simulink model "NAVI_V1_1"  (R2018a)
settings: Solver=VariableStepAuto  StartTime=0.0  StopTime=10.0  FixedStep=sampletime  RelTol=1e-3  EnableMultiTasking=on
PreLoadFcn:
  | NAVI_V1_BusInfo;
libraries: simulink x2
settings Model: Creator=IAEC nishito  LastModifiedBy=nishito
settings DataIOCC: LimitDataPoints=on  SaveFormat=Array  SignalLoggingSaveFormat=ModelDataLogs  SaveOutput=off
settings OptimizationCC: DefaultParameterBehavior=Inlined  ExpressionDepthLimit=2147483647  LifeSpan=inf
settings DebuggingCC: UnderspecifiedInitializationDetection=Classic  MergeDetectMultiDrivingBlocksExec=none  SolverPrmCheckMsg=warning  FcnCallInpInsideContextMsg=warning  StateNameClashWarn=warning  SFUnexpectedBacktrackingDiag=warning  SFNoUnconditionalDefaultTransitionDiag=warning  SFExecutionAtInitializationDiag=none
settings HardwareCC: ProdBitPerPointer=32  ProdBitPerSizeT=32  ProdBitPerPtrDiffT=32  ProdLargestAtomicFloat=None  ProdIntDivRoundTo=Undefined  ProdEndianess=Unspecified  ProdWordSize=32  ProdHWDeviceType=32-bit Generic
settings ModelReferenceCC: UpdateModelReferenceTargets=IfOutOfDate  PropagateSignalLabelsOutOfModel=off
settings CodeAppCC: StateflowObjectComments=on
settings GRTTargetCC: TargetLangStandard=C89/C90 (ANSI)  GeneratePreprocessorConditionals=Disable all  CombineOutputUpdateFcns=off  GRTInterface=on
settings ConfigComp: CovMetricSettings=dw  CovHtmlReporting=on  CovSaveCumulativeToWorkspaceVar=on  CovSaveSingleToWorkspaceVar=on  CovExternalEMLEnable=off  CovSFcnEnable=off

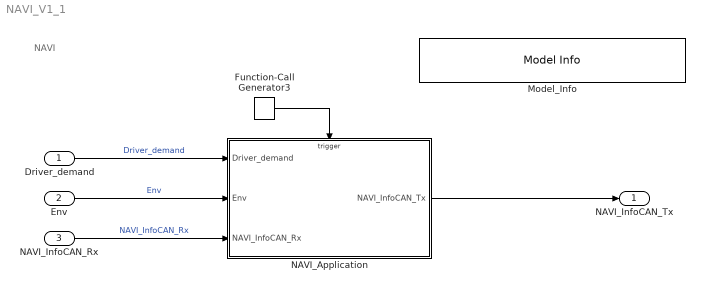
== system NAVI_V1_1 ==
  note: NAVI
  Driver_demand : Inport  OutDataTypeStr=Bus: Driver_demand_Bus
      settings: AttributesFormatString=<%<OutDataTypeStr>>
  Env : Inport  Port=2  OutDataTypeStr=Bus: Environment_Bus
      settings: AttributesFormatString=<%<OutDataTypeStr>>
  NAVI_InfoCAN_Rx : Inport  Port=3  OutDataTypeStr=Bus: NAVI_InfoCAN_Rx_Bus
      settings: AttributesFormatString=<%<OutDataTypeStr>>
  Function-Call Generator3 : simulink/Ports & Subsystems/Function-Call Generator  sample_time=0.1  numberOfIterations=1
      settings: AttributesFormatString=<sample_time=%<sample_time>>
  Model_Info : simulink/Model-Wide Utilities/Model Info  Frame=on  DisplayStringWithTags=|  HorizontalTextAlignment=Left  LeftAlignmentValue=0.02
      | Version  %<ModelVersion>
      | LastModifided by %<LastModifiedBy>  Date %<LastModificationDate>
      | Description  %<Description>
  NAVI_Application : Subsystem
  NAVI_InfoCAN_Tx : Outport  OutDataTypeStr=Bus: NAVI_InfoCAN_Tx_Bus
      settings: AttributesFormatString=<%<OutDataTypeStr>>
  wires:
  NAVI_Application/1(NAVI_InfoCAN_Tx) -> NAVI_InfoCAN_Tx/1
  NAVI_InfoCAN_Rx/1 -> NAVI_Application/3(NAVI_InfoCAN_Rx)  "NAVI_InfoCAN_Rx"
  Driver_demand/1 -> NAVI_Application/1(Driver_demand)  "Driver_demand"
  Function-Call Generator3/1 -> NAVI_Application/Trigger
  Env/1 -> NAVI_Application/2(Env)  "Env"

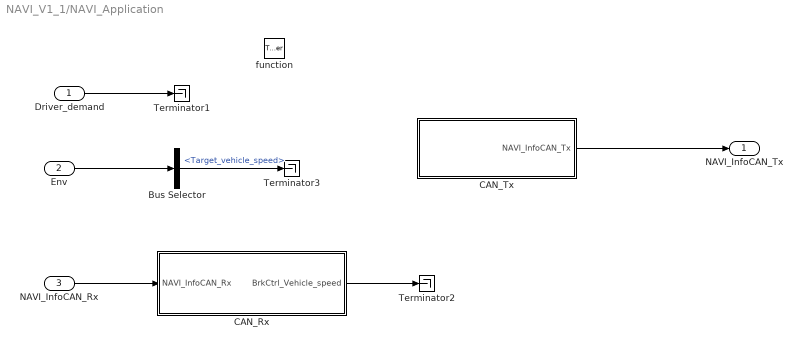
== system NAVI_V1_1/NAVI_Application ==
  Driver_demand : Inport
  Env : Inport  Port=2
  NAVI_InfoCAN_Rx : Inport  Port=3
  function : TriggerPort  TriggerType=function-call  VariantControl=Variant
  Bus Selector : BusSelector  OutputSignals=Target_vehicle_speed
  CAN_Rx : Subsystem
  CAN_Tx : Subsystem
  Terminator1 : Terminator
  Terminator2 : Terminator
  Terminator3 : Terminator
  NAVI_InfoCAN_Tx : Outport
  wires:
  Driver_demand/1 -> Terminator1/1
  NAVI_InfoCAN_Rx/1 -> CAN_Rx/1(NAVI_InfoCAN_Rx)
  CAN_Rx/1(BrkCtrl_Vehicle_speed) -> Terminator2/1
  Env/1 -> Bus Selector/1
  Bus Selector/1 -> Terminator3/1  "<Target_vehicle_speed>"
  CAN_Tx/1(NAVI_InfoCAN_Tx) -> NAVI_InfoCAN_Tx/1

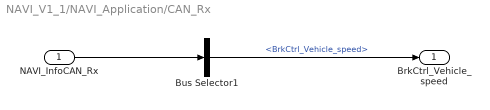
== system NAVI_V1_1/NAVI_Application/CAN_Rx ==
  NAVI_InfoCAN_Rx : Inport
  Bus Selector1 : BusSelector  OutputSignals=BrkCtrl_Vehicle_speed
  BrkCtrl_Vehicle_speed : Outport
  wires:
  NAVI_InfoCAN_Rx/1 -> Bus Selector1/1
  Bus Selector1/1 -> BrkCtrl_Vehicle_speed/1  "<BrkCtrl_Vehicle_speed>"

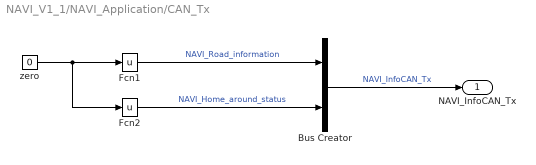
== system NAVI_V1_1/NAVI_Application/CAN_Tx ==
  Bus Creator : BusCreator  Inputs=2  OutDataTypeStr=Bus: NAVI_InfoCAN_Tx_Bus
      settings: AttributesFormatString=<%<OutDataTypeStr>>
  Fcn1 : Fcn  Expr=u
  Fcn2 : Fcn  Expr=u
  zero : Constant  Value=0
  NAVI_InfoCAN_Tx : Outport
  wires:
  Fcn1/1 -> Bus Creator/1  "NAVI_Road_information"
  zero/1 -> Fcn1/1, Fcn2/1
  Fcn2/1 -> Bus Creator/2  "NAVI_Home_around_status"
  Bus Creator/1 -> NAVI_InfoCAN_Tx/1  "NAVI_InfoCAN_Tx"
